simulink model "TClntDspl_DD"  (R2016b)
settings: configuration reference "CodeGenConfigSet" (kept outside this file)
values from neighbouring files (symbols this model uses):
  TClntDspl_bSwtPrs_C = Calibration.Parameter    [init_TClntDspl_DD.m]
  TClntDspl_O_P_ATS = Calibration.Parameter    [init_TClntDspl_DD.m]
  TClntDspl_PwmOut_swtBattCor_C = Calibration.Parameter    [init_TClntDspl_DD.m]
  TClntDspl_rCnv_CUR = Calibration.Parameter    [init_TClntDspl_DD.m]
  TClntDspl_rCnv_CURX = Calibration.Parameter    [init_TClntDspl_DD.m]
  TClntDspl_stEna_C = Calibration.Parameter    [init_TClntDspl_DD.m]
  TClntDspl_stPsDiaDisbl_C = Calibration.Parameter    [init_TClntDspl_DD.m]
  TClntDspl_stPsDisbl_C = Calibration.Parameter    [init_TClntDspl_DD.m]
  TClntDspl_tiPer_C = Calibration.Parameter    [init_TClntDspl_DD.m]
undefined symbols (not defined in the file or in its folder): Switch_conv
libraries: simulink x2
settings Model: Creator=Wei Liang  LastModifiedBy=Wei Liang
settings ConfigSetRef: SourceLocation=Base Workspace

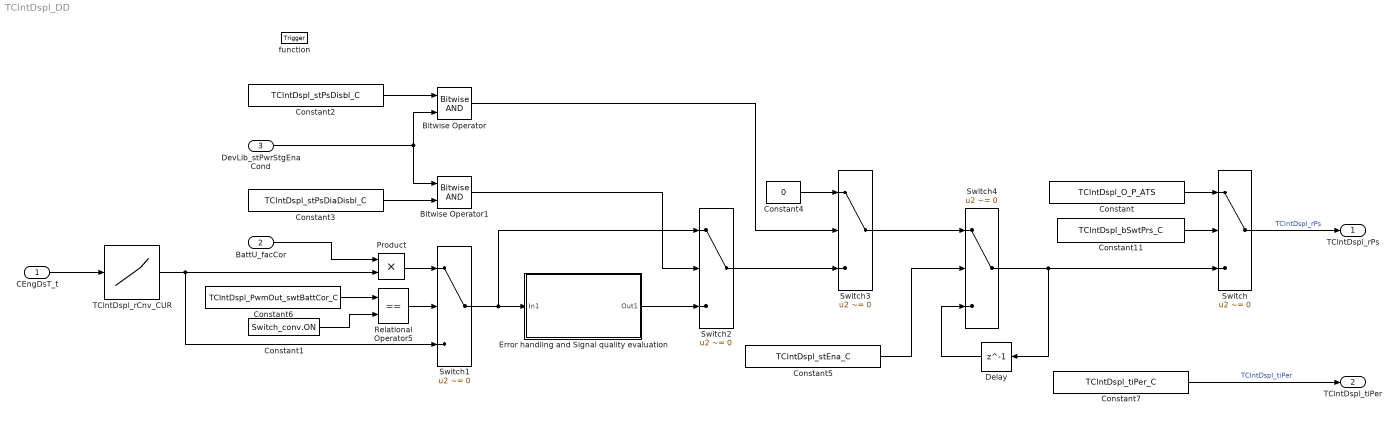
== system TClntDspl_DD ==
  CEngDsT_t : Inport  Tag=deg  Description=engine coolant temperature after filter  OutMin=-200  OutMax=200  OutDataTypeStr=Temp_deg
  BattU_facCor : Inport  Description=Battery correction factor  Port=2  OutMin=-32  OutMax=31.9  OutDataTypeStr=Factor
  DevLib_stPwrStgEnaCond : Inport  Description=Control unit status relevant to power stage deactivation/error diagnosis  Port=3  OutMin=0  OutMax=65535  OutDataTypeStr=State_uint16
  function : TriggerPort  TriggerType=function-call  VariantControl=Variant
  Bitwise Operator : simulink/Logic and Bit Operations/Bitwise Operator  logicop=AND  UseBitMask=off  NumInputPorts=2  BitMask=bin2dec('11011001')  BitMaskRealWorld=Stored Integer
  Bitwise Operator1 : simulink/Logic and Bit Operations/Bitwise Operator  logicop=AND  UseBitMask=off  NumInputPorts=2  BitMask=bin2dec('11011001')  BitMaskRealWorld=Stored Integer
  Constant : Constant  Value=TClntDspl_O_P_ATS
  Constant1 : Constant  Value=Switch_conv.ON  OutDataTypeStr=Inherit: Inherit via back propagation
  Constant11 : Constant  Value=TClntDspl_bSwtPrs_C  SampleTime=-1
  Constant2 : Constant  Value=TClntDspl_stPsDisbl_C
  Constant3 : Constant  Value=TClntDspl_stPsDiaDisbl_C
  Constant4 : Constant  Value=0  OutDataTypeStr=Inherit: Inherit via back propagation
  Constant5 : Constant  Value=TClntDspl_stEna_C
  Constant6 : Constant  Value=TClntDspl_PwmOut_swtBattCor_C
  Constant7 : Constant  Value=TClntDspl_tiPer_C  OutDataTypeStr=Time_PwmHigh_us  SampleTime=-1
  Delay : Delay  DelayLength=1  InitialCondition=0
  Error handling and Signal quality evaluation : Subsystem
  Product : Product  SaturateOnIntegerOverflow=on
  Relational Operator5 : RelationalOperator  Operator===  OutDataTypeStr=boolean  RndMeth=Simplest  InputSameDT=on
  Switch : Switch  Criteria=u2 ~= 0  OutDataTypeStr=Inherit: Inherit via back propagation
  Switch1 : Switch  Criteria=u2 ~= 0
  Switch2 : Switch  Criteria=u2 ~= 0  OutDataTypeStr=Inherit: Inherit via back propagation
  Switch3 : Switch  Criteria=u2 ~= 0  OutDataTypeStr=Inherit: Inherit via back propagation
  Switch4 : Switch  Criteria=u2 ~= 0
  TClntDspl_rCnv_CUR : Lookup_n-D  NumberOfTableDimensions=1  BreakpointsForDimension1=TClntDspl_rCnv_CURX  Table=TClntDspl_rCnv_CUR  ExtrapMethod=Clip  InternalRulePriority=Speed  RndMeth=Simplest
  TClntDspl_rPs : Outport  Tag=%  Description=Output to the power stage of coolant temperature PWM output to drive the gauge on the dashboard  OutMin=0  OutMax=100  OutDataTypeStr=DutyCycle_rate
  TClntDspl_tiPer : Outport  Tag=us  Description=Class Instance for PWM / Reference value for period duration (small type to limit dynamic range)  Port=2  OutMin=-107374182  OutMax=107374182  OutDataTypeStr=Time_PwmHigh_us
  wires:
  CEngDsT_t/1 -> TClntDspl_rCnv_CUR/1
  BattU_facCor/1 -> Product/1
  Product/1 -> Switch1/1
  TClntDspl_rCnv_CUR/1 -> Switch1/3, Product/2
  Switch1/1 -> Switch2/1, Error handling and Signal quality evaluation/1(In1)
  Error handling and Signal quality evaluation/1(Out1) -> Switch2/3
  Constant2/1 -> Bitwise Operator/1
  DevLib_stPwrStgEnaCond/1 -> Bitwise Operator1/1, Bitwise Operator/2
  Constant3/1 -> Bitwise Operator1/2
  Bitwise Operator1/1 -> Switch2/2
  Bitwise Operator/1 -> Switch3/2
  Switch2/1 -> Switch3/3
  Constant4/1 -> Switch3/1
  Switch3/1 -> Switch4/1
  Delay/1 -> Switch4/3
  Constant5/1 -> Switch4/2
  Switch4/1 -> Delay/1, Switch/3
  Constant/1 -> Switch/1
  Constant11/1 -> Switch/2
  Switch/1 -> TClntDspl_rPs/1  "TClntDspl_rPs"
  Constant1/1 -> Relational Operator5/2
  Relational Operator5/1 -> Switch1/2
  Constant6/1 -> Relational Operator5/1
  Constant7/1 -> TClntDspl_tiPer/1  "TClntDspl_tiPer"

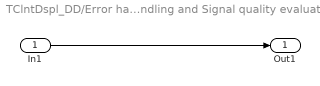
== system TClntDspl_DD/Error handling and Signal quality evaluation ==
  In1 : Inport
  Out1 : Outport
  wires:
  In1/1 -> Out1/1
